simulink model "Discrete"  (R2022b)
settings: Solver=ode45  StartTime=0.0  StopTime=10.0  MaxStep=.001  RelTol=1e-3  AbsTol=1e-6
undefined symbols (not defined in the file): B, fd, Ka, Kd, Ki, Kp, M, T, taua, v0, vref
settings Model: Creator=mcb  LastModifiedBy=ROG
settings SolverCC: AutoScaleAbsTol=off  AlgebraicLoopSolver=TrustRegion
settings DataIOCC: SaveFormat=Array  SignalLoggingSaveFormat=ModelDataLogs  SaveOutput=off  SaveTime=off  ReturnWorkspaceOutputs=off  TimeSaveName=time  SignalLoggingName=sigsOut
settings OptimizationCC: BooleanDataType=off  LifeSpan=inf
settings DebuggingCC: SaveWithParameterizedLinksMsg=none  UnderspecifiedInitializationDetection=Classic  MergeDetectMultiDrivingBlocksExec=none  SignalResolutionControl=TryResolveAllWithWarning  MultiTaskDSMMsg=warning  MultiTaskCondExecSysMsg=none  FcnCallInpInsideContextMsg=warning  UnconnectedInputMsg=warning  UnconnectedOutputMsg=warning  UnconnectedLineMsg=warning  SFUnexpectedBacktrackingDiag=warning  SFNoUnconditionalDefaultTransitionDiag=warning  SFExecutionAtInitializationDiag=none  SFMachineParentedDataDiag=warning  ArithmeticOperatorsInVariantConditions=warning
settings HardwareCC: ProdBitPerPointer=32  ProdBitPerSizeT=32  ProdBitPerPtrDiffT=32  ProdLargestAtomicFloat=None  ProdIntDivRoundTo=Undefined  ProdEndianess=Unspecified  ProdWordSize=32  ProdHWDeviceType=32-bit Generic  TargetUnknown=on
settings ModelReferenceCC: PropagateSignalLabelsOutOfModel=off
settings SFSimCC: SimUseLocalCustomCode=off  CustomCodeUndefinedFunction=UseInterfaceOnly
settings RTWCC: TemplateMakefile=grt_vc.tmf  RTWUseLocalCustomCode=off
settings CodeAppCC: StateflowObjectComments=on
settings GRTTargetCC: TargetLangStandard=C89/C90 (ANSI)  CombineOutputUpdateFcns=off  GRTInterface=on
settings ConfigComp: CovMetricSettings=dw  CovSaveCumulativeToWorkspaceVar=on  CovSaveSingleToWorkspaceVar=on  CovExternalEMLEnable=off  CovSFcnEnable=off

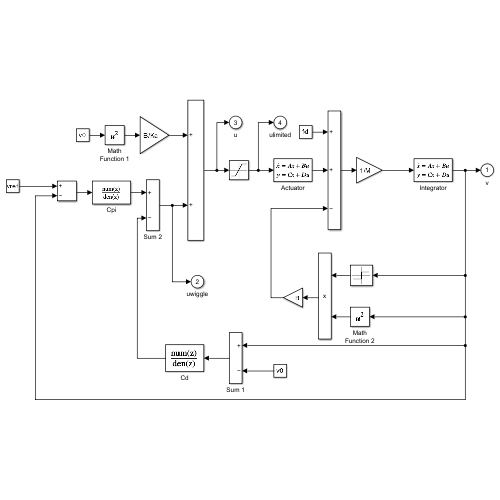
[thumbnail: Simulink's stored preview of the top-level diagram]
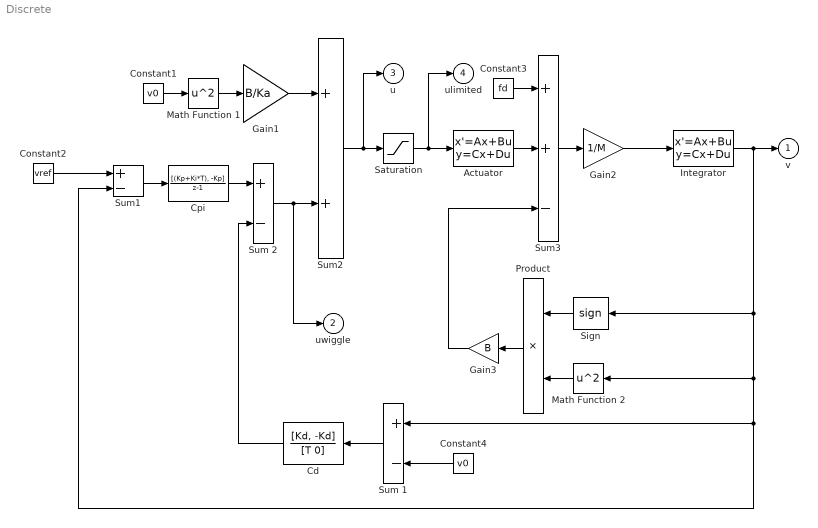
== system Discrete ==
  Actuator : StateSpace  A=-1/taua  B=Ka/taua  D=0  InitialCondition=B*v0^2
  Cd : DiscreteTransferFcn  Numerator=[Kd, -Kd]  Denominator=[T 0]  SampleTime=T
  Constant1 : Constant  Value=v0
  Constant2 : Constant  Value=vref
  Constant3 : Constant  Value=fd
  Constant4 : Constant  Value=v0
  Cpi : DiscreteTransferFcn  Numerator=[(Kp+Ki*T), -Kp]  Denominator=[1 -1]  SampleTime=T
  Gain1 : Gain  Gain=B/Ka  SaturateOnIntegerOverflow=on  OutDataTypeStr=Inherit: Same as input  ParamDataTypeStr=Inherit: Same as input
  Gain2 : Gain  Gain=1/M  SaturateOnIntegerOverflow=on  OutDataTypeStr=Inherit: Same as input  ParamDataTypeStr=Inherit: Same as input
  Gain3 : Gain  Gain=B  SaturateOnIntegerOverflow=on  OutDataTypeStr=Inherit: Same as input  ParamDataTypeStr=Inherit: Same as input
  Integrator : StateSpace  A=0  D=0  InitialCondition=v0
  Math Function 1 : Math  Operator=square  SignedPower=on
  Math Function 2 : Math  Operator=square  SignedPower=on
  Product : Product  InputSameDT=on  SaturateOnIntegerOverflow=on  OutDataTypeStr=Inherit: Same as first input
  Saturation : Saturate  UpperLimit=1  LowerLimit=0
  Sign : Signum
  Sum 1 : Sum  Inputs=+-  InputSameDT=on  SaturateOnIntegerOverflow=on  OutDataTypeStr=Inherit: Same as first input
  Sum 2 : Sum  Inputs=+-  InputSameDT=on  SaturateOnIntegerOverflow=on  OutDataTypeStr=Inherit: Same as first input
  Sum1 : Sum  Inputs=+-  InputSameDT=on  SaturateOnIntegerOverflow=on  OutDataTypeStr=Inherit: Same as first input
  Sum2 : Sum  InputSameDT=on  SaturateOnIntegerOverflow=on  OutDataTypeStr=Inherit: Same as first input
  Sum3 : Sum  Inputs=++-  InputSameDT=on  SaturateOnIntegerOverflow=on  OutDataTypeStr=Inherit: Same as first input
  v : Outport  InitialOutput=0
  uwiggle : Outport  Port=2  InitialOutput=0
  u : Outport  Port=3  InitialOutput=0
  ulimited : Outport  Port=4  InitialOutput=0
  wires:
  Constant2/1 -> Sum1/1
  Sum1/1 -> Cpi/1
  Sign/1 -> Product/1
  Math Function 2/1 -> Product/2
  Product/1 -> Gain3/1
  Gain3/1 -> Sum3/3
  Sum3/1 -> Gain2/1
  Sum2/1 -> Saturation/1, u/1
  Actuator/1 -> Sum3/2
  Saturation/1 -> Actuator/1, ulimited/1
  Cpi/1 -> Sum 2/1
  Gain1/1 -> Sum2/1
  Sum 2/1 -> Sum2/2, uwiggle/1
  Integrator/1 -> Sum 1/1, Sum1/2, Math Function 2/1, Sign/1, v/1
  Gain2/1 -> Integrator/1
  Math Function 1/1 -> Gain1/1
  Constant1/1 -> Math Function 1/1
  Constant3/1 -> Sum3/1
  Constant4/1 -> Sum 1/2
  Sum 1/1 -> Cd/1
  Cd/1 -> Sum 2/2
